simulink model "flash_3bit"  (R2021b)
settings: Solver=FixedStepDiscrete  StartTime=0.0  StopTime=5000*ts  FixedStep=ts  RelTol=1e-3
values from neighbouring files (symbols this model uses):
  fin = antismear(fin_pre,fs,nfft)    [launch_flash_3bit.m]
  ts = 1/fs    (= 1)    [launch_flash_3bit.m]
settings Model: Creator=umi  LastModifiedBy=DELL
settings SolverCC: AlgebraicLoopSolver=TrustRegion
settings DataIOCC: LimitDataPoints=on  SaveFormat=Array  SignalLoggingSaveFormat=ModelDataLogs  SaveOutput=off  SaveTime=off  ReturnWorkspaceOutputs=off
settings OptimizationCC: ExpressionDepthLimit=2147483647  LifeSpan=inf
settings DebuggingCC: UnderspecifiedInitializationDetection=Classic  MergeDetectMultiDrivingBlocksExec=none  SolverPrmCheckMsg=warning  FcnCallInpInsideContextMsg=warning  StateNameClashWarn=warning  SFUnexpectedBacktrackingDiag=warning  SFNoUnconditionalDefaultTransitionDiag=warning  SFExecutionAtInitializationDiag=none  SFMachineParentedDataDiag=warning  ArithmeticOperatorsInVariantConditions=warning
settings HardwareCC: ProdBitPerPointer=32  ProdBitPerSizeT=32  ProdBitPerPtrDiffT=32  ProdLargestAtomicFloat=None  ProdIntDivRoundTo=Undefined  ProdEndianess=Unspecified  ProdWordSize=32  ProdHWDeviceType=32-bit Generic
settings ModelReferenceCC: PropagateSignalLabelsOutOfModel=off
settings SFSimCC: SimUseLocalCustomCode=off  CustomCodeUndefinedFunction=UseInterfaceOnly
settings RTWCC: RTWUseLocalCustomCode=off
settings CodeAppCC: StateflowObjectComments=on
settings GRTTargetCC: TargetLangStandard=C89/C90 (ANSI)  CombineOutputUpdateFcns=off  GRTInterface=on
settings ConfigComp: CovMetricSettings=dw  CovSaveCumulativeToWorkspaceVar=on  CovSaveSingleToWorkspaceVar=on  CovExternalEMLEnable=off  CovSFcnEnable=off

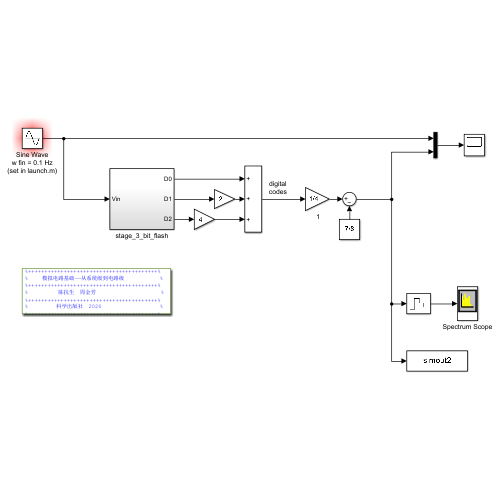
[thumbnail: Simulink's stored preview of the top-level diagram]
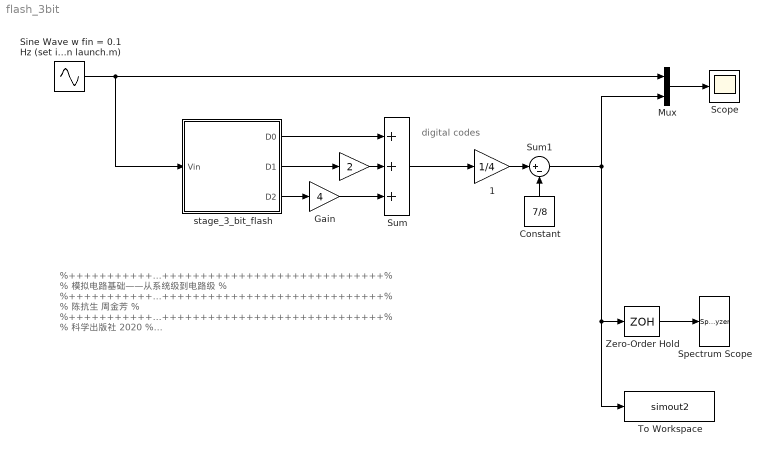
== system flash_3bit ==
  note: digital
      | codes
  note: %++++++++++++++++++++++++++++++++++++++++%
      | % 模拟电路基础——从系统级到电路级 %
      | %++++++++++++++++++++++++++++++++++++++++%
      | % 陈抗生 周金芳 %
      | %++++++++++++++++++++++++++++++++++++++++%
      | % 科学出版社 2020 %
      | %++++++++++++++++++++++++++++++++++++++++%
  " " : Gain  Gain=2
  " 1" : Gain  Gain=1/4
  Constant : Constant  Value=7/8
  Gain : Gain  Gain=4
  Mux : Mux  Inputs=2
  Scope : Scope
  Sine Wave w fin = 0.1 Hz (set in launch.m) : Sin  Frequency=2*pi*fin  SampleTime=0
  Spectrum Scope : SpectrumAnalyzer
  Sum : Sum  Inputs=+++
  Sum1 : Sum  Inputs=|+-
  To Workspace : ToWorkspace  VariableName=simout2  SampleTime=-1
  Zero-Order Hold : ZeroOrderHold
  stage_3_bit_flash : Subsystem
  wires:
  stage_3_bit_flash/1(D0) -> Sum/1
  stage_3_bit_flash/2(D1) -> " "/1
  stage_3_bit_flash/3(D2) -> Gain/1
  Mux/1 -> Scope/1
  " "/1 -> Sum/2
  Sine Wave w fin = 0.1 Hz (set in launch.m)/1 -> stage_3_bit_flash/1(Vin), Mux/1
  Gain/1 -> Sum/3
  " 1"/1 -> Sum1/1
  Constant/1 -> Sum1/2
  Sum1/1 -> To Workspace/1, Zero-Order Hold/1, Mux/2
  Zero-Order Hold/1 -> Spectrum Scope/1
  Sum/1 -> " 1"/1

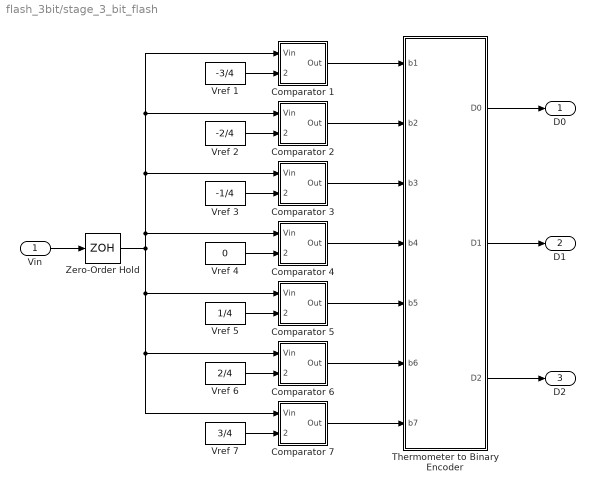
== system flash_3bit/stage_3_bit_flash ==
  Vin : Inport
  Comparator 1 : Subsystem
  Comparator 2 : Subsystem
  Comparator 3 : Subsystem
  Comparator 4 : Subsystem
  Comparator 5 : Subsystem
  Comparator 6 : Subsystem
  Comparator 7 : Subsystem
  Thermometer to Binary Encoder : Subsystem
  Vref 1 : Constant  Value=-3/4
  Vref 2 : Constant  Value=-2/4
  Vref 3 : Constant  Value=-1/4
  Vref 4 : Constant  Value=0
  Vref 5 : Constant  Value=1/4
  Vref 6 : Constant  Value=2/4
  Vref 7 : Constant  Value=3/4
  Zero-Order Hold : ZeroOrderHold  SampleTime=ts
  D0 : Outport
  D1 : Outport  Port=2
  D2 : Outport  Port=3
  wires:
  Vin/1 -> Zero-Order Hold/1
  Vref 1/1 -> Comparator 1/2(Vref)
  Thermometer to Binary Encoder/1(D0) -> D0/1
  Thermometer to Binary Encoder/2(D1) -> D1/1
  Thermometer to Binary Encoder/3(D2) -> D2/1
  Comparator 1/1(Out) -> Thermometer to Binary Encoder/1(b1)
  Vref 2/1 -> Comparator 2/2(Vref)
  Comparator 2/1(Out) -> Thermometer to Binary Encoder/2(b2)
  Vref 3/1 -> Comparator 3/2(Vref)
  Comparator 3/1(Out) -> Thermometer to Binary Encoder/3(b3)
  Vref 4/1 -> Comparator 4/2(Vref)
  Comparator 4/1(Out) -> Thermometer to Binary Encoder/4(b4)
  Vref 5/1 -> Comparator 5/2(Vref)
  Comparator 5/1(Out) -> Thermometer to Binary Encoder/5(b5)
  Vref 6/1 -> Comparator 6/2(Vref)
  Comparator 6/1(Out) -> Thermometer to Binary Encoder/6(b6)
  Vref 7/1 -> Comparator 7/2(Vref)
  Comparator 7/1(Out) -> Thermometer to Binary Encoder/7(b7)
  Zero-Order Hold/1 -> Comparator 4/1(Vin), Comparator 3/1(Vin), Comparator 2/1(Vin), Comparator 1/1(Vin), Comparator 5/1(Vin), Comparator 7/1(Vin), Comparator 6/1(Vin)

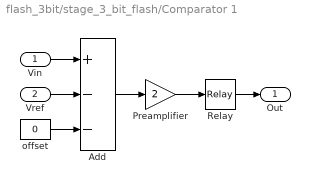
== system flash_3bit/stage_3_bit_flash/Comparator 1 ==
  Vin : Inport
  Vref : Inport  Port=2
  Add : Sum  Inputs=+--
  Preamplifier : Gain  Gain=2
  Relay : Relay  OnSwitchValue=0  OffSwitchValue=0
  offset : Constant  Value=0
  Out : Outport
  wires:
  Vin/1 -> Add/1
  Relay/1 -> Out/1
  Vref/1 -> Add/2
  Preamplifier/1 -> Relay/1
  Add/1 -> Preamplifier/1
  offset/1 -> Add/3

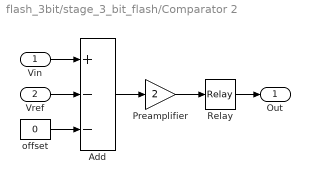
== system flash_3bit/stage_3_bit_flash/Comparator 2 ==
  Vin : Inport
  Vref : Inport  Port=2
  Add : Sum  Inputs=+--
  Preamplifier : Gain  Gain=2
  Relay : Relay  OnSwitchValue=0  OffSwitchValue=0
  offset : Constant  Value=0
  Out : Outport
  wires:
  Vin/1 -> Add/1
  Relay/1 -> Out/1
  Vref/1 -> Add/2
  Preamplifier/1 -> Relay/1
  Add/1 -> Preamplifier/1
  offset/1 -> Add/3

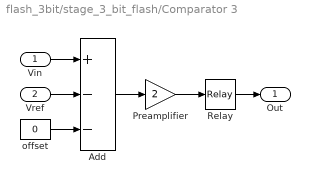
== system flash_3bit/stage_3_bit_flash/Comparator 3 ==
  Vin : Inport
  Vref : Inport  Port=2
  Add : Sum  Inputs=+--
  Preamplifier : Gain  Gain=2
  Relay : Relay  OnSwitchValue=0  OffSwitchValue=0
  offset : Constant  Value=0
  Out : Outport
  wires:
  Vin/1 -> Add/1
  Relay/1 -> Out/1
  Vref/1 -> Add/2
  Preamplifier/1 -> Relay/1
  Add/1 -> Preamplifier/1
  offset/1 -> Add/3

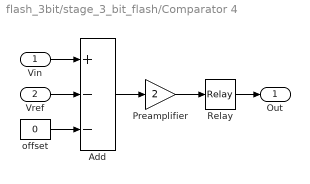
== system flash_3bit/stage_3_bit_flash/Comparator 4 ==
  Vin : Inport
  Vref : Inport  Port=2
  Add : Sum  Inputs=+--
  Preamplifier : Gain  Gain=2
  Relay : Relay  OnSwitchValue=0  OffSwitchValue=0
  offset : Constant  Value=0
  Out : Outport
  wires:
  Vin/1 -> Add/1
  Relay/1 -> Out/1
  Vref/1 -> Add/2
  Preamplifier/1 -> Relay/1
  Add/1 -> Preamplifier/1
  offset/1 -> Add/3

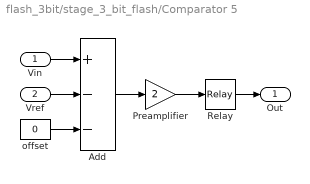
== system flash_3bit/stage_3_bit_flash/Comparator 5 ==
  Vin : Inport
  Vref : Inport  Port=2
  Add : Sum  Inputs=+--
  Preamplifier : Gain  Gain=2
  Relay : Relay  OnSwitchValue=0  OffSwitchValue=0
  offset : Constant  Value=0
  Out : Outport
  wires:
  Vin/1 -> Add/1
  Relay/1 -> Out/1
  Vref/1 -> Add/2
  Preamplifier/1 -> Relay/1
  Add/1 -> Preamplifier/1
  offset/1 -> Add/3

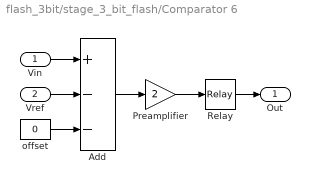
== system flash_3bit/stage_3_bit_flash/Comparator 6 ==
  Vin : Inport
  Vref : Inport  Port=2
  Add : Sum  Inputs=+--
  Preamplifier : Gain  Gain=2
  Relay : Relay  OnSwitchValue=0  OffSwitchValue=0
  offset : Constant  Value=0
  Out : Outport
  wires:
  Vin/1 -> Add/1
  Relay/1 -> Out/1
  Vref/1 -> Add/2
  Preamplifier/1 -> Relay/1
  Add/1 -> Preamplifier/1
  offset/1 -> Add/3

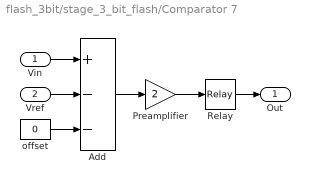
== system flash_3bit/stage_3_bit_flash/Comparator 7 ==
  Vin : Inport
  Vref : Inport  Port=2
  Add : Sum  Inputs=+--
  Preamplifier : Gain  Gain=2
  Relay : Relay  OnSwitchValue=0  OffSwitchValue=0
  offset : Constant  Value=0
  Out : Outport
  wires:
  Vin/1 -> Add/1
  Relay/1 -> Out/1
  Vref/1 -> Add/2
  Preamplifier/1 -> Relay/1
  Add/1 -> Preamplifier/1
  offset/1 -> Add/3

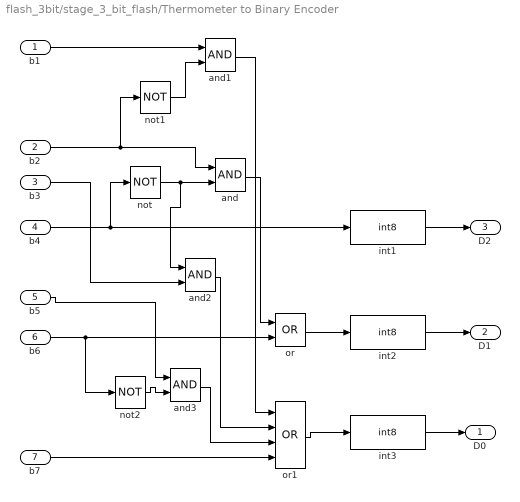
== system flash_3bit/stage_3_bit_flash/Thermometer to Binary Encoder ==
  b1 : Inport
  b2 : Inport  Port=2
  b3 : Inport  Port=3
  b4 : Inport  Port=4
  b5 : Inport  Port=5
  b6 : Inport  Port=6
  b7 : Inport  Port=7
  and{,1..3} (4 alike) : Logic  AllPortsSameDT=off  OutDataTypeStr=boolean
  int1 : DataTypeConversion  OutDataTypeStr=int8
  int2 : DataTypeConversion  OutDataTypeStr=int8
  int3 : DataTypeConversion  OutDataTypeStr=int8
  not : Logic  Operator=NOT  AllPortsSameDT=off  OutDataTypeStr=boolean
  not1 : Logic  Operator=NOT  AllPortsSameDT=off  OutDataTypeStr=boolean
  not2 : Logic  Operator=NOT  AllPortsSameDT=off  OutDataTypeStr=boolean
  or : Logic  Operator=OR  AllPortsSameDT=off  OutDataTypeStr=boolean
  or1 : Logic  Operator=OR  Inputs=4  AllPortsSameDT=off  OutDataTypeStr=boolean
  D0 : Outport
  D1 : Outport  Port=2
  D2 : Outport  Port=3
  wires:
  b4/1 -> not/1, int1/1
  not/1 -> and/2, and2/1
  b2/1 -> and/1, not1/1
  b6/1 -> or/2, not2/1
  and/1 -> or/1
  or/1 -> int2/1
  or1/1 -> int3/1
  b1/1 -> and1/1
  not1/1 -> and1/2
  and1/1 -> or1/1
  b3/1 -> and2/2
  and2/1 -> or1/2
  b7/1 -> or1/4
  not2/1 -> and3/2
  b5/1 -> and3/1
  int2/1 -> D1/1
  int3/1 -> D0/1
  and3/1 -> or1/3
  int1/1 -> D2/1
